simulink model "Local_trajectory_export"  (R2021a)
settings: configuration reference "AION_IDS_Speedgoat" (kept outside this file)
undefined symbols (not defined in the file): LATERAL_DISTANCE_THRESHOLD, MAX_GLOBAL_TRAJECTORY_WAY_POINT_NUMBER, MAX_LOCAL_TRAJECTORY_WAY_POINT_NUMBER, MAX_TRAJECTORY_LENGTH, START_END_DISTANCE_THRESHOLD
libraries: simulink x1
(part 2 of 2)

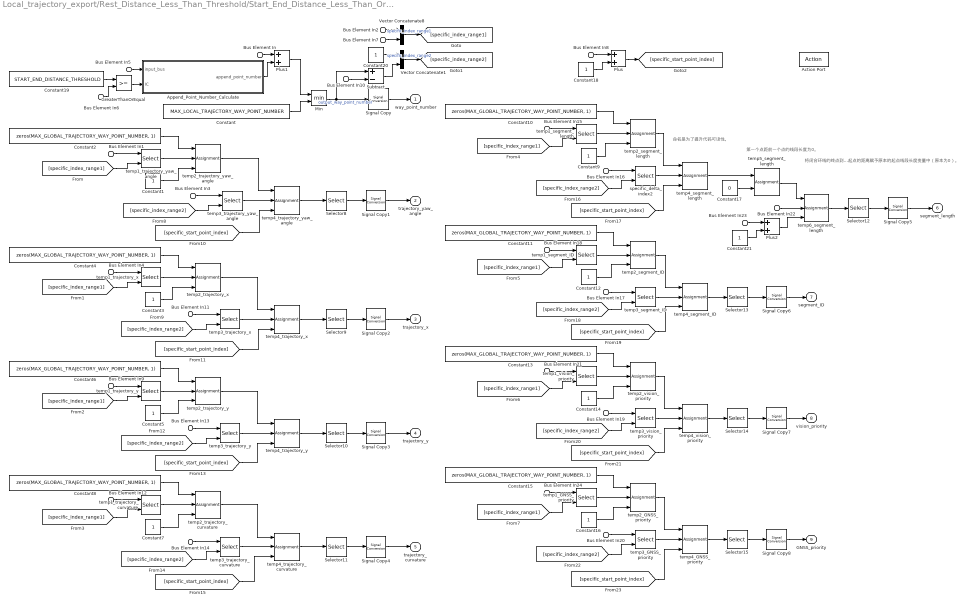
== system Local_trajectory_export/Rest_Distance_Less_Than_Threshold/Start_End_Distance_Less_Than_Or_Equal_Threshold ==
  note: 将闭合环线的终点到起点的距离赋予原本的起点线段长度变量中（原本为0）。
  note: 第一个点距前一个点的线段长度为0。
  note: 命名是为了提升代码可读性。
  Bus Element In5 : Inport  PortName=input_bus
  Bus Element In{,8,10,23} (4 alike) : Inport  PortName=input_bus  Element=rest_point_number
  Bus Element In1 : Inport  PortName=input_bus  Element=global_trajectory_yaw_angle
  Bus Element In3 : Inport  PortName=input_bus  Element=global_trajectory_yaw_angle
  Bus Element In2 : Inport  PortName=input_bus  Element=closest_segment_start_point_index_current
  Bus Element In4 : Inport  PortName=input_bus  Element=global_trajectory_x
  Bus Element In11 : Inport  PortName=input_bus  Element=global_trajectory_x
  Bus Element In9 : Inport  PortName=input_bus  Element=global_trajectory_y
  Bus Element In13 : Inport  PortName=input_bus  Element=global_trajectory_y
  Bus Element In12 : Inport  PortName=input_bus  Element=global_trajectory_curvature
  Bus Element In14 : Inport  PortName=input_bus  Element=global_trajectory_curvature
  Bus Element In15 : Inport  PortName=input_bus  Element=global_trajectory_segment_length
  Bus Element In16 : Inport  PortName=input_bus  Element=global_trajectory_segment_length
  Bus Element In18 : Inport  PortName=input_bus  Element=global_trajectory_segment_ID
  Bus Element In17 : Inport  PortName=input_bus  Element=global_trajectory_segment_ID
  Bus Element In21 : Inport  PortName=input_bus  Element=global_trajectory_vision_priority
  Bus Element In19 : Inport  PortName=input_bus  Element=global_trajectory_vision_priority
  Bus Element In24 : Inport  PortName=input_bus  Element=global_trajectory_GNSS_priority
  Bus Element In20 : Inport  PortName=input_bus  Element=global_trajectory_GNSS_priority
  Bus Element In6 : Inport  PortName=input_bus  Element=start_end_distance
  Bus Element In22 : Inport  PortName=input_bus  Element=start_end_distance
  Bus Element In7 : Inport  PortName=input_bus  Element=global_trajectory_point_number
  Action Port : ActionPort  PropagateVarSize=During execution  ActionPortLabel=else
  Append_Point_Number_Calculate : Subsystem  Description=遍历搜索满足导出轨迹累计弧长条件的从闭合环线起点往后接续在从最近点到终点的局部轨迹之后的点数。  TreatAsAtomicUnit=on
  Constant : Constant  Value=MAX_LOCAL_TRAJECTORY_WAY_POINT_NUMBER  VectorParams1D=off  OutDataTypeStr=int32  SampleTime=-1
  Constant{1,3,5,7,9,12,14,16,18,20..21} (11 alike) : Constant  OutDataTypeStr=int32  SampleTime=-1
  Constant{2,4,6,8,10} (5 alike) : Constant  Value=zeros(MAX_GLOBAL_TRAJECTORY_WAY_POINT_NUMBER, 1)  OutDataTypeStr=double  SampleTime=-1
  Constant11 : Constant  Value=zeros(MAX_GLOBAL_TRAJECTORY_WAY_POINT_NUMBER, 1)  OutDataTypeStr=int8  SampleTime=-1
  Constant13 : Constant  Value=zeros(MAX_GLOBAL_TRAJECTORY_WAY_POINT_NUMBER, 1)  OutDataTypeStr=int8  SampleTime=-1
  Constant15 : Constant  Value=zeros(MAX_GLOBAL_TRAJECTORY_WAY_POINT_NUMBER, 1)  OutDataTypeStr=int8  SampleTime=-1
  Constant17 : Constant  Value=0  OutDataTypeStr=double  SampleTime=-1
  Constant19 : Constant  Value=START_END_DISTANCE_THRESHOLD  OutDataTypeStr=double  SampleTime=-1
  GreaterThanOrEqual : RelationalOperator  OutDataTypeStr=boolean  RndMeth=Simplest
  Min : MinMax  Inputs=2  OutDataTypeStr=int32
  Plus : Sum
  Plus1 : Sum
  Plus2 : Sum
  Selector{8..15} (8 alike) : Selector  IndexOptions=Starting index (dialog)  Indices=1  OutputSizes=MAX_LOCAL_TRAJECTORY_WAY_POINT_NUMBER
  Signal Copy{,1..8} (9 alike) : SignalConversion  OverrideOpt=off
  Subtract : Sum  Inputs=+-
  Vector Concatenate1 : Concatenate
  Vector Concatenate8 : Concatenate
  specific_delta_index2 : Selector  IndexOptions=Starting and ending indices (port)  Indices=[1 3]  OutputSizes=MAX_LOCAL_TRAJECTORY_WAY_POINT_NUMBER
  temp1_GNSS_priority : Selector  IndexOptions=Starting and ending indices (port)  Indices=[1 3]  OutputSizes=MAX_LOCAL_TRAJECTORY_WAY_POINT_NUMBER
  temp1_segment_ID : Selector  IndexOptions=Starting and ending indices (port)  Indices=[1 3]  OutputSizes=MAX_LOCAL_TRAJECTORY_WAY_POINT_NUMBER
  temp1_segment_length : Selector  IndexOptions=Starting and ending indices (port)  Indices=[1 3]  OutputSizes=MAX_LOCAL_TRAJECTORY_WAY_POINT_NUMBER
  temp1_trajectory_curvature : Selector  IndexOptions=Starting and ending indices (port)  Indices=[1 3]  OutputSizes=MAX_LOCAL_TRAJECTORY_WAY_POINT_NUMBER
  temp1_trajectory_x : Selector  IndexOptions=Starting and ending indices (port)  Indices=[1 3]  OutputSizes=MAX_LOCAL_TRAJECTORY_WAY_POINT_NUMBER
  temp1_trajectory_y : Selector  IndexOptions=Starting and ending indices (port)  Indices=[1 3]  OutputSizes=MAX_LOCAL_TRAJECTORY_WAY_POINT_NUMBER
  temp1_trajectory_yaw_angle : Selector  IndexOptions=Starting and ending indices (port)  Indices=[1 3]  OutputSizes=MAX_LOCAL_TRAJECTORY_WAY_POINT_NUMBER
  temp1_vision_priority : Selector  IndexOptions=Starting and ending indices (port)  Indices=[1 3]  OutputSizes=MAX_LOCAL_TRAJECTORY_WAY_POINT_NUMBER
  temp2_GNSS_priority : Assignment  DiagnosticForDimensions=Warning  IndexOptions=Starting index (port)  Indices=1  OutputSizes=MAX_LOCAL_TRAJECTORY_WAY_POINT_NUMBER
  temp2_segment_ID : Assignment  DiagnosticForDimensions=Warning  IndexOptions=Starting index (port)  Indices=1  OutputSizes=MAX_LOCAL_TRAJECTORY_WAY_POINT_NUMBER
  temp2_segment_length : Assignment  DiagnosticForDimensions=Warning  IndexOptions=Starting index (port)  Indices=1  OutputSizes=MAX_LOCAL_TRAJECTORY_WAY_POINT_NUMBER
  temp2_trajectory_curvature : Assignment  DiagnosticForDimensions=Warning  IndexOptions=Starting index (port)  Indices=1  OutputSizes=MAX_LOCAL_TRAJECTORY_WAY_POINT_NUMBER
  temp2_trajectory_x : Assignment  DiagnosticForDimensions=Warning  IndexOptions=Starting index (port)  Indices=1  OutputSizes=MAX_LOCAL_TRAJECTORY_WAY_POINT_NUMBER
  temp2_trajectory_y : Assignment  DiagnosticForDimensions=Warning  IndexOptions=Starting index (port)  Indices=1  OutputSizes=MAX_LOCAL_TRAJECTORY_WAY_POINT_NUMBER
  temp2_trajectory_yaw_angle : Assignment  DiagnosticForDimensions=Warning  IndexOptions=Starting index (port)  Indices=1  OutputSizes=MAX_LOCAL_TRAJECTORY_WAY_POINT_NUMBER
  temp2_vision_priority : Assignment  DiagnosticForDimensions=Warning  IndexOptions=Starting index (port)  Indices=1  OutputSizes=MAX_LOCAL_TRAJECTORY_WAY_POINT_NUMBER
  temp3_GNSS_priority : Selector  IndexOptions=Starting and ending indices (port)  Indices=[1 3]  OutputSizes=MAX_LOCAL_TRAJECTORY_WAY_POINT_NUMBER
  temp3_segment_ID : Selector  IndexOptions=Starting and ending indices (port)  Indices=[1 3]  OutputSizes=MAX_LOCAL_TRAJECTORY_WAY_POINT_NUMBER
  temp3_trajectory_curvature : Selector  IndexOptions=Starting and ending indices (port)  Indices=[1 3]  OutputSizes=MAX_LOCAL_TRAJECTORY_WAY_POINT_NUMBER
  temp3_trajectory_x : Selector  IndexOptions=Starting and ending indices (port)  Indices=[1 3]  OutputSizes=MAX_LOCAL_TRAJECTORY_WAY_POINT_NUMBER
  temp3_trajectory_y : Selector  IndexOptions=Starting and ending indices (port)  Indices=[1 3]  OutputSizes=MAX_LOCAL_TRAJECTORY_WAY_POINT_NUMBER
  temp3_trajectory_yaw_angle : Selector  IndexOptions=Starting and ending indices (port)  Indices=[1 3]  OutputSizes=MAX_LOCAL_TRAJECTORY_WAY_POINT_NUMBER
  temp3_vision_priority : Selector  IndexOptions=Starting and ending indices (port)  Indices=[1 3]  OutputSizes=MAX_LOCAL_TRAJECTORY_WAY_POINT_NUMBER
  temp4_GNSS_priority : Assignment  DiagnosticForDimensions=Warning  IndexOptions=Starting index (port)  Indices=1  OutputSizes=MAX_LOCAL_TRAJECTORY_WAY_POINT_NUMBER
  temp4_segment_ID : Assignment  DiagnosticForDimensions=Warning  IndexOptions=Starting index (port)  Indices=1  OutputSizes=MAX_LOCAL_TRAJECTORY_WAY_POINT_NUMBER
  temp4_segment_length : Assignment  DiagnosticForDimensions=Warning  IndexOptions=Starting index (port)  Indices=1  OutputSizes=MAX_LOCAL_TRAJECTORY_WAY_POINT_NUMBER
  temp4_trajectory_curvature : Assignment  DiagnosticForDimensions=Warning  IndexOptions=Starting index (port)  Indices=1  OutputSizes=MAX_LOCAL_TRAJECTORY_WAY_POINT_NUMBER
  temp4_trajectory_x : Assignment  DiagnosticForDimensions=Warning  IndexOptions=Starting index (port)  Indices=1  OutputSizes=MAX_LOCAL_TRAJECTORY_WAY_POINT_NUMBER
  temp4_trajectory_y : Assignment  DiagnosticForDimensions=Warning  IndexOptions=Starting index (port)  Indices=1  OutputSizes=MAX_LOCAL_TRAJECTORY_WAY_POINT_NUMBER
  temp4_trajectory_yaw_angle : Assignment  DiagnosticForDimensions=Warning  IndexOptions=Starting index (port)  Indices=1  OutputSizes=MAX_LOCAL_TRAJECTORY_WAY_POINT_NUMBER
  temp4_vision_priority : Assignment  DiagnosticForDimensions=Warning  IndexOptions=Starting index (port)  Indices=1  OutputSizes=MAX_LOCAL_TRAJECTORY_WAY_POINT_NUMBER
  temp5_segment_length : Assignment  Description=第一个点距前一个点的线段长度为0。  OutputInitialize=Specify size for each dimension in table  DiagnosticForDimensions=Warning  IndexOptions=Index vector (dialog)  Indices=1  OutputSizes=MAX_LOCAL_TRAJECTORY_WAY_POINT_NUMBER
  temp6_segment_length : Assignment  Description=将闭合环线的终点到起点的距离赋予原本的起点线段长度变量中（原本为0）。  DiagnosticForDimensions=Warning  IndexOptions=Index vector (port)  Indices=1  OutputSizes=MAX_LOCAL_TRAJECTORY_WAY_POINT_NUMBER
  way_point_number : Outport  Description=导出的局部轨迹有效路点个数，自然数，无量纲。  OutDataTypeStr=int32  PortDimensions=1
  trajectory_yaw_angle : Outport  Description=导出的局部轨迹横摆角数组，有效数据数量为way_point_number，其余补零，实数，deg。  Port=2  OutDataTypeStr=double  PortDimensions=MAX_LOCAL_TRAJECTORY_WAY_POINT_NUMBER
  trajectory_x : Outport  Description=导出的局部轨迹x坐标数组，有效数据数量为way_point_number，其余补零，实数，m。  Port=3  OutDataTypeStr=double  PortDimensions=MAX_LOCAL_TRAJECTORY_WAY_POINT_NUMBER
  trajectory_y : Outport  Description=导出的局部轨迹y坐标数组，有效数据数量为way_point_number，其余补零，实数，m。  Port=4  OutDataTypeStr=double  PortDimensions=MAX_LOCAL_TRAJECTORY_WAY_POINT_NUMBER
  trajectory_curvature : Outport  Description=导出的局部轨迹曲率数组，有效数据数量为way_point_number，其余补零，实数，1/m。  Port=5  OutDataTypeStr=double  PortDimensions=MAX_LOCAL_TRAJECTORY_WAY_POINT_NUMBER
  segment_length : Outport  Description=导出的局部轨迹路点到前一个点的线段长度数组，有效数据数量为way_point_number，其余补零，正实数，m。  Port=6  OutDataTypeStr=double  PortDimensions=MAX_LOCAL_TRAJECTORY_WAY_POINT_NUMBER
  segment_ID : Outport  Description=导出的局部轨迹区间代号数组，有效数据数量为way_point_number，其余补零，正整数，无量纲。  Port=7  OutDataTypeStr=int8  PortDimensions=MAX_LOCAL_TRAJECTORY_WAY_POINT_NUMBER
  vision_priority : Outport  Description=导出的局部轨迹视觉循迹优先级数组，有效数据数量为way_point_number，其余补零，自然数，无量纲。  Port=8  OutDataTypeStr=int8  PortDimensions=MAX_LOCAL_TRAJECTORY_WAY_POINT_NUMBER
  GNSS_priority : Outport  Description=导出的局部轨迹GNSS循迹优先级数组，有效数据数量为way_point_number，其余补零，自然数，无量纲。  Port=9  OutDataTypeStr=int8  PortDimensions=MAX_LOCAL_TRAJECTORY_WAY_POINT_NUMBER
  wires:
  temp2_GNSS_priority/1 -> temp4_GNSS_priority/1
  Constant15/1 -> temp2_GNSS_priority/1
  temp1_GNSS_priority/1 -> temp2_GNSS_priority/2
  [specific_index_range1] -> temp1_GNSS_priority/2
  temp2_vision_priority/1 -> temp4_vision_priority/1
  Constant13/1 -> temp2_vision_priority/1
  temp1_vision_priority/1 -> temp2_vision_priority/2
  [specific_index_range1] -> temp1_vision_priority/2
  Bus Element In21/1 -> temp1_vision_priority/1
  temp2_segment_ID/1 -> temp4_segment_ID/1
  Constant11/1 -> temp2_segment_ID/1
  temp1_segment_ID/1 -> temp2_segment_ID/2
  [specific_index_range1] -> temp1_segment_ID/2
  Selector12/1 -> Signal Copy5/1
  temp5_segment_length/1 -> temp6_segment_length/1
  Constant17/1 -> temp5_segment_length/2
  temp2_segment_length/1 -> temp4_segment_length/1
  Constant10/1 -> temp2_segment_length/1
  temp1_segment_length/1 -> temp2_segment_length/2
  [specific_index_range1] -> temp1_segment_length/2
  Selector11/1 -> Signal Copy4/1
  temp2_trajectory_curvature/1 -> temp4_trajectory_curvature/1
  Constant8/1 -> temp2_trajectory_curvature/1
  [specific_index_range1] -> temp1_trajectory_curvature/2
  temp2_trajectory_y/1 -> temp4_trajectory_y/1
  Selector10/1 -> Signal Copy3/1
  Constant6/1 -> temp2_trajectory_y/1
  [specific_index_range1] -> temp1_trajectory_y/2
  Constant4/1 -> temp2_trajectory_x/1
  Constant3/1 -> temp2_trajectory_x/3
  temp1_trajectory_x/1 -> temp2_trajectory_x/2
  [specific_index_range1] -> temp1_trajectory_x/2
  Constant2/1 -> temp2_trajectory_yaw_angle/1
  Constant1/1 -> temp2_trajectory_yaw_angle/3
  temp1_trajectory_yaw_angle/1 -> temp2_trajectory_yaw_angle/2
  [specific_index_range1] -> temp1_trajectory_yaw_angle/2
  Vector Concatenate8/1 -> [specific_index_range1]  "specific_index_range1"
  Bus Element In2/1 -> Vector Concatenate8/1
  Selector13/1 -> Signal Copy6/1
  Selector14/1 -> Signal Copy7/1
  Selector9/1 -> Signal Copy2/1
  temp2_trajectory_yaw_angle/1 -> temp4_trajectory_yaw_angle/1
  Selector15/1 -> Signal Copy8/1
  Bus Element In24/1 -> temp1_GNSS_priority/1
  Constant16/1 -> temp2_GNSS_priority/3
  Constant14/1 -> temp2_vision_priority/3
  Bus Element In18/1 -> temp1_segment_ID/1
  Constant12/1 -> temp2_segment_ID/3
  Constant9/1 -> temp2_segment_length/3
  Bus Element In15/1 -> temp1_segment_length/1
  Bus Element In12/1 -> temp1_trajectory_curvature/1
  temp1_trajectory_curvature/1 -> temp2_trajectory_curvature/2
  Constant7/1 -> temp2_trajectory_curvature/3
  Constant5/1 -> temp2_trajectory_y/3
  temp1_trajectory_y/1 -> temp2_trajectory_y/2
  Bus Element In9/1 -> temp1_trajectory_y/1
  Bus Element In4/1 -> temp1_trajectory_x/1
  Bus Element In1/1 -> temp1_trajectory_yaw_angle/1
  Min/1 -> Subtract/1, Signal Copy/1  "output_way_point_number"
  Constant/1 -> Min/2
  Bus Element In5/1 -> Append_Point_Number_Calculate/1(input_bus)
  Bus Element In/1 -> Plus1/1
  Append_Point_Number_Calculate/1(append_point_number) -> Plus1/2
  Plus1/1 -> Min/1
  Constant19/1 -> GreaterThanOrEqual/1
  Bus Element In6/1 -> GreaterThanOrEqual/2
  GreaterThanOrEqual/1 -> Append_Point_Number_Calculate/2(IC)
  Bus Element In7/1 -> Vector Concatenate8/2
  Constant20/1 -> Vector Concatenate1/1
  Vector Concatenate1/1 -> [specific_index_range2]  "specific_index_range2"
  Bus Element In10/1 -> Subtract/2
  Subtract/1 -> Vector Concatenate1/2
  Bus Element In3/1 -> temp3_trajectory_yaw_angle/1
  [specific_index_range2] -> temp3_trajectory_yaw_angle/2
  temp3_trajectory_yaw_angle/1 -> temp4_trajectory_yaw_angle/2
  Constant18/1 -> Plus/2
  Bus Element In8/1 -> Plus/1
  temp4_trajectory_yaw_angle/1 -> Selector8/1
  Bus Element In11/1 -> temp3_trajectory_x/1
  [specific_index_range2] -> temp3_trajectory_x/2
  temp3_trajectory_x/1 -> temp4_trajectory_x/2
  [specific_start_point_index] -> temp4_trajectory_x/3
  Plus/1 -> [specific_start_point_index]
  [specific_start_point_index] -> temp4_trajectory_yaw_angle/3
  temp2_trajectory_x/1 -> temp4_trajectory_x/1
  temp4_trajectory_x/1 -> Selector9/1
  Bus Element In13/1 -> temp3_trajectory_y/1
  temp3_trajectory_y/1 -> temp4_trajectory_y/2
  [specific_start_point_index] -> temp4_trajectory_y/3
  [specific_index_range2] -> temp3_trajectory_y/2
  temp4_trajectory_y/1 -> Selector10/1
  [specific_start_point_index] -> temp4_trajectory_curvature/3
  temp3_trajectory_curvature/1 -> temp4_trajectory_curvature/2
  Bus Element In14/1 -> temp3_trajectory_curvature/1
  [specific_index_range2] -> temp3_trajectory_curvature/2
  temp4_trajectory_curvature/1 -> Selector11/1
  Bus Element In16/1 -> specific_delta_index2/1
  [specific_start_point_index] -> temp4_segment_length/3
  [specific_index_range2] -> specific_delta_index2/2
  specific_delta_index2/1 -> temp4_segment_length/2
  temp4_segment_length/1 -> temp5_segment_length/1
  [specific_start_point_index] -> temp4_segment_ID/3
  [specific_index_range2] -> temp3_segment_ID/2
  temp3_segment_ID/1 -> temp4_segment_ID/2
  Bus Element In17/1 -> temp3_segment_ID/1
  temp4_segment_ID/1 -> Selector13/1
  [specific_start_point_index] -> temp4_vision_priority/3
  Bus Element In19/1 -> temp3_vision_priority/1
  [specific_index_range2] -> temp3_vision_priority/2
  temp3_vision_priority/1 -> temp4_vision_priority/2
  temp4_vision_priority/1 -> Selector14/1
  [specific_start_point_index] -> temp4_GNSS_priority/3
  Bus Element In20/1 -> temp3_GNSS_priority/1
  [specific_index_range2] -> temp3_GNSS_priority/2
  temp3_GNSS_priority/1 -> temp4_GNSS_priority/2
  temp4_GNSS_priority/1 -> Selector15/1
  Selector8/1 -> Signal Copy1/1
  Signal Copy/1 -> way_point_number/1
  Signal Copy1/1 -> trajectory_yaw_angle/1
  Signal Copy2/1 -> trajectory_x/1
  Signal Copy3/1 -> trajectory_y/1
  Signal Copy4/1 -> trajectory_curvature/1
  Signal Copy5/1 -> segment_length/1
  Signal Copy6/1 -> segment_ID/1
  Signal Copy7/1 -> vision_priority/1
  Signal Copy8/1 -> GNSS_priority/1
  Bus Element In22/1 -> temp6_segment_length/2
  Bus Element In23/1 -> Plus2/1
  Constant21/1 -> Plus2/2
  Plus2/1 -> temp6_segment_length/3
  temp6_segment_length/1 -> Selector12/1

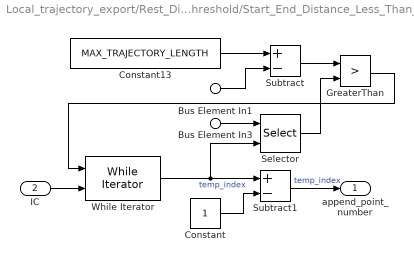
== system Local_trajectory_export/Rest_Distance_Less_Than_Threshold/Start_End_Distance_Less_Than_Or_Equal_Threshold/Append_Point_Number_Calculate ==
  Bus Element In3 : Inport  PortName=input_bus  Element=global_trajectory_cumulative_length
  Bus Element In1 : Inport  PortName=input_bus  Element=rest_distance
  IC : Inport  Port=2
  Constant : Constant  OutDataTypeStr=int32  SampleTime=-1
  Constant13 : Constant  Value=MAX_TRAJECTORY_LENGTH  OutDataTypeStr=double  SampleTime=-1
  GreaterThan : RelationalOperator  Operator=>  OutDataTypeStr=boolean  RndMeth=Simplest
  Selector : Selector  IndexOptions=Index vector (port)  Indices=[1 3]  OutputSizes=1
  Subtract : Sum  Inputs=+-
  Subtract1 : Sum  Inputs=+-
  While Iterator : WhileIterator  MaxIters=MAX_GLOBAL_TRAJECTORY_WAY_POINT_NUMBER  ResetStates=reset  ShowIterationPort=on
  append_point_number : Outport  Description=从闭合环线起点往后接续在从最近点到终点的局部轨迹之后的点数。  OutDataTypeStr=int32
  wires:
  IC/1 -> While Iterator/2
  Bus Element In3/1 -> Selector/1
  While Iterator/1 -> Subtract1/1, Selector/2  "temp_index"
  Constant13/1 -> Subtract/1
  Bus Element In1/1 -> Subtract/2
  Subtract/1 -> GreaterThan/1
  Selector/1 -> GreaterThan/2
  GreaterThan/1 -> While Iterator/1
  Constant/1 -> Subtract1/2
  Subtract1/1 -> append_point_number/1  "temp_index"
